simulink model "KiemChungDH"  (R2022a)
settings: Solver=VariableStepAuto  StartTime=0.0  StopTime=10.0  RelTol=1e-3
libraries: simulink_extras x4
settings Model: Creator=Vũ Quốc Khánh  LastModifiedBy=Vũ Quốc Khánh

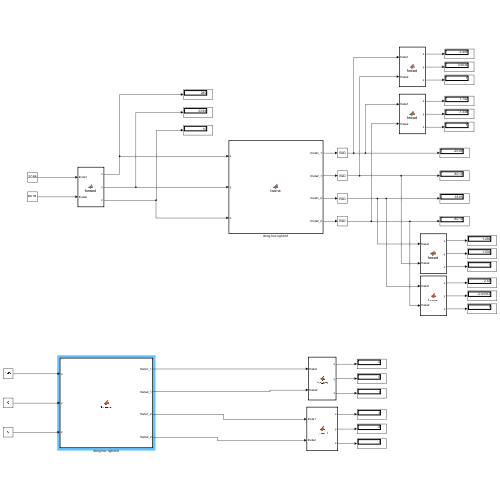
[thumbnail: Simulink's stored preview of the top-level diagram]
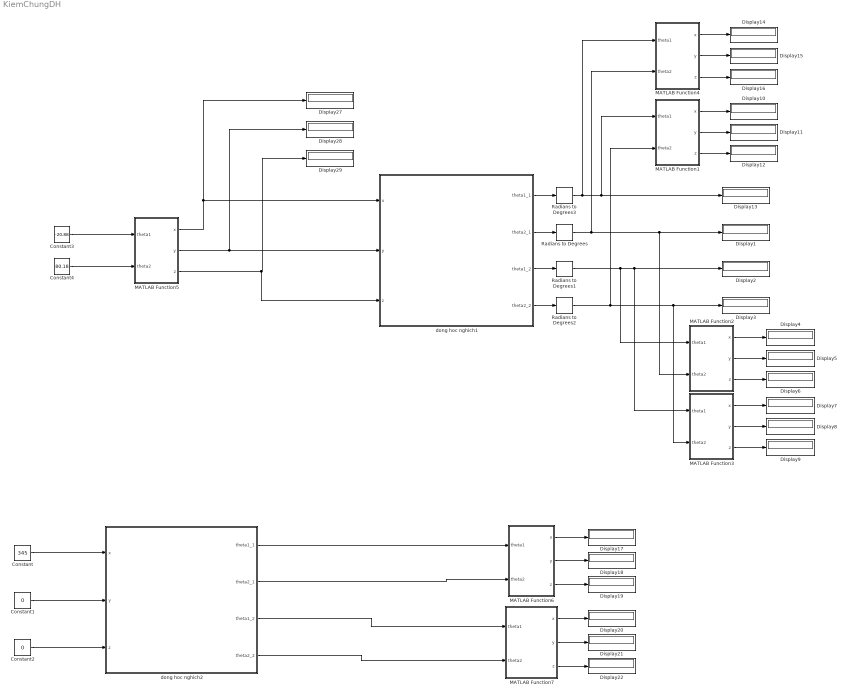
== system KiemChungDH ==
  Constant : Constant  Value=345
  Constant1 : Constant  Value=0
  Constant2 : Constant  Value=0
  Constant3 : Constant  Value=-20.88
  Constant4 : Constant  Value=80.18
  Display{1..22,27..29} (25 alike) : Display
  MATLAB Function1 : MATLAB Function  TreatAsAtomicUnit=on
  MATLAB Function2 : MATLAB Function  TreatAsAtomicUnit=on
  MATLAB Function3 : MATLAB Function  TreatAsAtomicUnit=on
  MATLAB Function4 : MATLAB Function  TreatAsAtomicUnit=on
  MATLAB Function5 : MATLAB Function  TreatAsAtomicUnit=on
  MATLAB Function6 : MATLAB Function  TreatAsAtomicUnit=on
  MATLAB Function7 : MATLAB Function  TreatAsAtomicUnit=on
  Radians to Degrees{,1..3} (4 alike) : simulink_extras/Transformations/Radians to Degrees
  dong hoc nghich1 : MATLAB Function  TreatAsAtomicUnit=on
  dong hoc nghich2 : MATLAB Function  TreatAsAtomicUnit=on
  wires:
  Constant3/1 -> MATLAB Function5/1(theta1)
  Constant4/1 -> MATLAB Function5/2(theta2)
  Radians to Degrees2/1 -> MATLAB Function1/2(theta2), MATLAB Function3/2(theta2), Display3/1
  Radians to Degrees1/1 -> MATLAB Function2/1(theta1), MATLAB Function3/1(theta1), Display2/1
  dong hoc nghich1/2(theta2_1) -> Radians to Degrees/1
  dong hoc nghich1/1(theta1_1) -> Radians to Degrees3/1
  Radians to Degrees/1 -> MATLAB Function4/2(theta2), MATLAB Function2/2(theta2), Display1/1
  dong hoc nghich1/4(theta2_2) -> Radians to Degrees2/1
  MATLAB Function5/3(z) -> dong hoc nghich1/3(z), Display29/1
  MATLAB Function5/1(x) -> dong hoc nghich1/1(x), Display27/1
  MATLAB Function5/2(y) -> dong hoc nghich1/2(y), Display28/1
  MATLAB Function2/1(x) -> Display4/1
  MATLAB Function2/2(y) -> Display5/1
  MATLAB Function2/3(z) -> Display6/1
  MATLAB Function3/1(x) -> Display7/1
  MATLAB Function3/2(y) -> Display8/1
  MATLAB Function3/3(z) -> Display9/1
  MATLAB Function1/1(x) -> Display10/1
  MATLAB Function1/2(y) -> Display11/1
  MATLAB Function1/3(z) -> Display12/1
  MATLAB Function4/3(z) -> Display16/1
  MATLAB Function4/2(y) -> Display15/1
  MATLAB Function4/1(x) -> Display14/1
  dong hoc nghich1/3(theta1_2) -> Radians to Degrees1/1
  Radians to Degrees3/1 -> MATLAB Function4/1(theta1), Display13/1, MATLAB Function1/1(theta1)
  dong hoc nghich2/1(theta1_1) -> MATLAB Function6/1(theta1)
  dong hoc nghich2/2(theta2_1) -> MATLAB Function6/2(theta2)
  dong hoc nghich2/4(theta2_2) -> MATLAB Function7/2(theta2)
  dong hoc nghich2/3(theta1_2) -> MATLAB Function7/1(theta1)
  Constant/1 -> dong hoc nghich2/1(x)
  Constant1/1 -> dong hoc nghich2/2(y)
  Constant2/1 -> dong hoc nghich2/3(z)
  MATLAB Function6/1(x) -> Display17/1
  MATLAB Function6/2(y) -> Display18/1
  MATLAB Function6/3(z) -> Display19/1
  MATLAB Function7/2(y) -> Display21/1
  MATLAB Function7/3(z) -> Display22/1
  MATLAB Function7/1(x) -> Display20/1

== matlab function KiemChungDH/MATLAB Function6 ==
  data: theta1 input; x output; theta2 input; y output; z output
function [x,y,z] = forward(theta1,theta2)
%% Khai bao bien
l1=1;
l2=1;
l3=1;
d=1;
x=l1 + l2*cosd(theta1) + l3* ((cosd(theta1)*cosd(theta2))-sind(theta1)*sind(theta2));
%y= cosd(q1)*l3*sind(q2) + sind(q1)*(l2+l3*cosd(q2));
y=l2*sind(theta1) + l3*sind(theta1+theta2);
z=d;
%%diem dau cuoi

== matlab function KiemChungDH/MATLAB Function7 ==
  data: theta1 input; x output; theta2 input; y output; z output
function [x,y,z] = forward(theta1,theta2)
%% Khai bao bien
l1=1;
l2=1;
l3=1;
d=1;
x=l1 + l2*cosd(theta1) + l3* ((cosd(theta1)*cosd(theta2))-sind(theta1)*sind(theta2));
%y= cosd(q1)*l3*sind(q2) + sind(q1)*(l2+l3*cosd(q2));
y=l2*sind(theta1) + l3*sind(theta1+theta2);
z=d;
%%diem dau cuoi

== matlab function KiemChungDH/MATLAB Function1 ==
  data: theta1 input; x output; theta2 input; y output; z output
function [x,y,z] = forward(theta1,theta2)
%% Khai bao bien
l1=1;
l2=1;
l3=1;
d=1;
x=l1 + l2*cosd(theta1) + l3* ((cosd(theta1)*cosd(theta2))-sind(theta1)*sind(theta2));
%y= cosd(q1)*l3*sind(q2) + sind(q1)*(l2+l3*cosd(q2));
y=l2*sind(theta1) + l3*sind(theta1+theta2);
z=d;
%%diem dau cuoi

== matlab function KiemChungDH/MATLAB Function2 ==
  data: theta1 input; x output; theta2 input; y output; z output
function [x,y,z] = forward(theta1,theta2)
%% Khai bao bien
l1=1;
l2=1;
l3=1;
d=1;
x=l1 + l2*cosd(theta1) + l3* ((cosd(theta1)*cosd(theta2))-sind(theta1)*sind(theta2));
%y= cosd(q1)*l3*sind(q2) + sind(q1)*(l2+l3*cosd(q2));
y=l2*sind(theta1) + l3*sind(theta1+theta2);
z=d;
%%diem dau cuoi

== matlab function KiemChungDH/MATLAB Function3 ==
  data: theta1 input; x output; theta2 input; y output; z output
function [x,y,z] = forward(theta1,theta2)
%% Khai bao bien
l1=1;
l2=1;
l3=1;
d=1;
x=l1 + l2*cosd(theta1) + l3* ((cosd(theta1)*cosd(theta2))-sind(theta1)*sind(theta2));
%y= cosd(q1)*l3*sind(q2) + sind(q1)*(l2+l3*cosd(q2));
y=l2*sind(theta1) + l3*sind(theta1+theta2);
z=d;
%%diem dau cuoi

== matlab function KiemChungDH/MATLAB Function4 ==
  data: theta1 input; x output; theta2 input; y output; z output
function [x,y,z] = forward(theta1,theta2)
%% Khai bao bien
l1=1;
l2=1;
l3=1;
d=1;
x=l1 + l2*cosd(theta1) + l3* ((cosd(theta1)*cosd(theta2))-sind(theta1)*sind(theta2));
%y= cosd(q1)*l3*sind(q2) + sind(q1)*(l2+l3*cosd(q2));
y=l2*sind(theta1) + l3*sind(theta1+theta2);
z=d;
%%diem dau cuoi

== matlab function KiemChungDH/dong hoc nghich2 ==
  data: x input; theta1_1 output; y input; z input; theta2_1 output; theta1_2 output; theta2_2 output
%%function [theta1, theta2] = Inverse(x,y,z)
    %%L1=1; 
   %% L2=1; 
    %%L3=1;
        %% theta2:
    %%c2=((x-L1)^2+y^2-L3^2-L1^2)/(2*L2*L3);
    % Bo nghiem 1
    %%for i=1:2
   %%     if i==1
     %%     s2=sqrt(1-c2^2);
    %%    else
   %%       s2=-sqrt(1-c2^2);
   %% end
    %%theta2=atan2(s2,c2);
   %% c1=((x-L1)*(L3*cos(theta2)+L2)+y*L3*sin(theta2))/((L3*cos(theta2)+L2)*(L3*cos(theta2)+L2)+(L3*sin(theta2))^2);
    %%s1=((L3*cos(theta2)+L2)*y -(x-L1)*L3*sin(theta2))/((L3*cos(theta2)+L2)*(L3*cos(theta2)+L2)+(L3*sin(theta2))^2);
    %%fprintf('Bo nghiem: %d ',i);
    %%theta2
    %%theta1=atan2(s1,c1)
    %%d=z

function [theta1_1, theta2_1, theta1_2, theta2_2] = Inverse(x, y, z)
    
    % Định nghĩa các hằng số
    L1 = 65; 
    L2 = 170; 
    L3 = 110;

    % Tính c2 cho theta2
    c2 = ((x - L1)^2 + y^2 - L3^2 - L2^2) / (2 * L2 * L3);
    

    % Khởi tạo các biến đầu ra cho các nghiệm
    theta1 = zeros(1, 2);
    theta2 = zeros(1, 2);
    
    for i = 1:2
        % Chọn giá trị phù hợp cho s2
        if i == 1
            s2 = sqrt(1 - c2^2);
        else
            s2 = -sqrt(1 - c2^2);
        end
        
        % Tính theta2 dựa vào s2 và c2
        theta2(i) = atan2(s2, c2);
        
        % Tính theta1 dựa vào theta2
        c1 = ((x - L1) * (L3 * cos(theta2(i)) + L2) + y * L3 * sin(theta2(i))) / ...
             ((L3 * cos(theta2(i)) + L2)^2 + (L3 * sin(theta2(i)))^2);
        s1 = ((L3 * cos(theta2(i)) + L2) * y - (x - L1) * L3 * sin(theta2(i))) / ...
             ((L3 * cos(theta2(i)) + L2)^2 + (L3 * sin(theta2(i)))^2);
        
        % Tính theta1
        theta1(i) = atan2(s1, c1);
        
        % Hiển thị kết quả
        %fprintf('Nghiệm %d: theta1 = %.4f, theta2 = %.4f\n', i, theta1(i), theta2(i));
    end
    
    % Gán các giá trị đầu ra tương ứng với hai bộ nghiệm
    theta1_1 = theta1(1);
    theta2_1 = theta2(1);
    theta1_2 = theta1(2);
    theta2_2 = theta2(2);
end

== matlab function KiemChungDH/dong hoc nghich1 ==
  data: x input; theta1_1 output; y input; z input; theta2_1 output; theta1_2 output; theta2_2 output
%%function [theta1, theta2] = Inverse(x,y,z)
    %%L1=1; 
   %% L2=1; 
    %%L3=1;
        %% theta2:
    %%c2=((x-L1)^2+y^2-L3^2-L1^2)/(2*L2*L3);
    % Bo nghiem 1
    %%for i=1:2
   %%     if i==1
     %%     s2=sqrt(1-c2^2);
    %%    else
   %%       s2=-sqrt(1-c2^2);
   %% end
    %%theta2=atan2(s2,c2);
   %% c1=((x-L1)*(L3*cos(theta2)+L2)+y*L3*sin(theta2))/((L3*cos(theta2)+L2)*(L3*cos(theta2)+L2)+(L3*sin(theta2))^2);
    %%s1=((L3*cos(theta2)+L2)*y -(x-L1)*L3*sin(theta2))/((L3*cos(theta2)+L2)*(L3*cos(theta2)+L2)+(L3*sin(theta2))^2);
    %%fprintf('Bo nghiem: %d ',i);
    %%theta2
    %%theta1=atan2(s1,c1)
    %%d=z

function [theta1_1, theta2_1, theta1_2, theta2_2] = Inverse(x, y, z)
    
    % Định nghĩa các hằng số
    L1 = 65; 
    L2 = 170; 
    L3 = 110;

    % Tính c2 cho theta2
    c2 = ((x - L1)^2 + y^2 - L3^2 - L2^2) / (2 * L2 * L3);
    

    % Khởi tạo các biến đầu ra cho các nghiệm
    theta1 = zeros(1, 2);
    theta2 = zeros(1, 2);
    
    for i = 1:2
        % Chọn giá trị phù hợp cho s2
        if i == 1
            s2 = sqrt(1 - c2^2);
        else
            s2 = -sqrt(1 - c2^2);
        end
        
        % Tính theta2 dựa vào s2 và c2
        theta2(i) = atan2(s2, c2);
        
        % Tính theta1 dựa vào theta2
        c1 = ((x - L1) * (L3 * cos(theta2(i)) + L2) + y * L3 * sin(theta2(i))) / ...
             ((L3 * cos(theta2(i)) + L2)^2 + (L3 * sin(theta2(i)))^2);
        s1 = ((L3 * cos(theta2(i)) + L2) * y - (x - L1) * L3 * sin(theta2(i))) / ...
             ((L3 * cos(theta2(i)) + L2)^2 + (L3 * sin(theta2(i)))^2);
        
        % Tính theta1
        theta1(i) = atan2(s1, c1);
        
        % Hiển thị kết quả
        %fprintf('Nghiệm %d: theta1 = %.4f, theta2 = %.4f\n', i, theta1(i), theta2(i));
    end
    
    % Gán các giá trị đầu ra tương ứng với hai bộ nghiệm
    theta1_1 = theta1(1);
    theta2_1 = theta2(1);
    theta1_2 = theta1(2);
    theta2_2 = theta2(2);
end

== matlab function KiemChungDH/MATLAB Function5 ==
  data: theta1 input; x output; theta2 input; y output; z output
function [x,y,z] = forward(theta1,theta2)
%% Khai bao bien
l1=65;
l2=170;
l3=110;
d=10;
%x=l1 + l2*cosd(theta1) + l3* ((cosd(theta1)*cosd(theta2))-sind(theta1)*sind(theta2));
x=l1 + l2*cosd(theta1) + l3* (cosd(theta1+theta2));
%y= cosd(q1)*l3*sind(q2) + sind(q1)*(l2+l3*cosd(q2));
y=l2*sind(theta1) + l3*sind(theta1+theta2);
z=d;
%%diem dau cuoi
